simulink model "controller_v13"  (R2020b)
settings: Solver=ode4  StartTime=0.0  StopTime=inf  RelTol=1e-3
undefined symbols (not defined in the file): ctr, DiscIntNeverNeededParam, flt, IO397, mdl, rbt, rsim, som, ukf_P0_flat, ukf_prediction_time, ukf_s0, ukf_sys, ukf_use_prediction
libraries: simulink x31, slrealtimeloglib x5, slrealtimeseriallib x5, speedgoatlib_fpga_analog_io x4, slrealtimetgmanagement x3, speedgoatlib_fpga x2, speedgoatlib_fpga_dio x1, slrealtimeutilitieslib x1
(part 3 of 5)

== system controller_v13/signal generator/Drive_Signal4/AveragedAmp_filtered ==
  note: To avoid having signal "jump",
      | we want SMOOTH transitions
      | in frequency (i.e., a weighted sum
      | of current freq and freq some delta t ago)
  note: time constant 0.002sec
      | for 10kHz samping
  In1 : Inport
  Discrete Transfer Fcn : DiscreteTransferFcn  Numerator=[0.05]  Denominator=[1 -.95]
  Out1 : Outport
  wires:
  In1/1 -> Discrete Transfer Fcn/1
  Discrete Transfer Fcn/1 -> Out1/1

== system controller_v13/signal generator/Drive_Signal4/AveragedOffset_filtered ==
  note: To avoid having signal "jump",
      | we want SMOOTH transitions
      | in frequency (i.e., a weighted sum
      | of current freq and freq some delta t ago)
  note: c
  note: time constant 0.02sec
      | for 10kHz samping
  In1 : Inport
  Discrete Transfer Fcn : DiscreteTransferFcn  Numerator=[0.05]  Denominator=[1 -.95]
  Out1 : Outport
  wires:
  In1/1 -> Discrete Transfer Fcn/1
  Discrete Transfer Fcn/1 -> Out1/1

== system controller_v13/signal generator/Drive_Signal4/AveragedTau_filtered ==
  note: To avoid having signal "jump",
      | we want SMOOTH transitions
      | in frequency (i.e., a weighted sum
      | of current freq and freq some delta t ago)
  note: time constant 0.002sec
      | for 10kHz samping
  In1 : Inport
  Discrete Transfer Fcn : DiscreteTransferFcn  Numerator=[0.05]  Denominator=[1, -0.95]
  Out1 : Outport
  wires:
  In1/1 -> Discrete Transfer Fcn/1
  Discrete Transfer Fcn/1 -> Out1/1

== system controller_v13/signal generator/Drive_Signal4/SignalForRamp_binary ==
  note: Should output 1 or -1,
      | so signal ramps UP to 1
      | or DOWN to 0.
  In1 : Inport
  Add : Sum  Inputs=+-
  Compare To Zero : simulink/Logic and Bit Operations/Compare To Zero  relop=>  OutDataTypeStr=uint8  ZeroCross=off
  Constant : Constant
  Data Type Conversion : DataTypeConversion  OutDataTypeStr=double
  Gain : Gain  Gain=2
  Out1 : Outport
  wires:
  In1/1 -> Compare To Zero/1
  Compare To Zero/1 -> Data Type Conversion/1
  Gain/1 -> Add/1
  Constant/1 -> Add/2
  Add/1 -> Out1/1
  Data Type Conversion/1 -> Gain/1

== system controller_v13/signal generator/Drive_Signal4/SignalForSin_binary ==
  note: We want this to stay "high" for 1
      | second after the actual "enable"
      | is turned off...
  In1 : Inport
  Compare To Zero : simulink/Logic and Bit Operations/Compare To Zero  relop=>  OutDataTypeStr=uint8  ZeroCross=off
  Data Type Conversion : DataTypeConversion  OutDataTypeStr=double
  Out1 : Outport
  wires:
  In1/1 -> Compare To Zero/1
  Compare To Zero/1 -> Data Type Conversion/1
  Data Type Conversion/1 -> Out1/1

== system controller_v13/signal generator/Drive_Signal4/Subsystem ==
  note: positive value pushes the left wing forward
  split cycle mu : Inport
  In2 : Inport  Port=2
  1-mu : Sum  Inputs=+-
  2f : Gain  Gain=2
  2nd harmonic : Trigonometry  OutputSignalType=real
  2pi : Gain  Gain=2*pi
  Abs1 : Abs
  Add : Sum
  Constant : Constant
  combined sines : Sum
  deg to rad : Gain  Gain=pi/180
  f : Gain  Gain=-1
  first harmonic : Trigonometry  OutputSignalType=real
  omega*t : DiscreteIntegrator  SampleTime=-1  ICPrevOutput=DiscIntNeverNeededParam  ICPrevScaledInput=DiscIntNeverNeededParam
  phase offset : Constant  Value=0
  signal with gain1 : Product  RndMeth=Zero
  signal with gain2 : Product  RndMeth=Zero
  split cycle signal : Outport
  wires:
  2f/1 -> 2nd harmonic/1
  first harmonic/1 -> signal with gain1/2
  Constant/1 -> 1-mu/1
  split cycle mu/1 -> f/1, Abs1/1
  1-mu/1 -> signal with gain1/1
  2nd harmonic/1 -> signal with gain2/2
  signal with gain1/1 -> combined sines/1
  signal with gain2/1 -> combined sines/2
  combined sines/1 -> split cycle signal/1
  f/1 -> signal with gain2/1
  Abs1/1 -> 1-mu/2
  In2/1 -> 2pi/1
  2pi/1 -> omega*t/1
  omega*t/1 -> Add/2
  Add/1 -> first harmonic/1, 2f/1
  phase offset/1 -> deg to rad/1
  deg to rad/1 -> Add/1

== system controller_v13/Adaptive Controller/adaptive system/integrator/safety2 ==
  In1 : Inport
  Compare To Constant1 : simulink/Logic and Bit Operations/Compare To Constant  relop=<=  const=inf  OutDataTypeStr=uint8
  Switch1 : Switch  Threshold=0.5
  zero1 : Constant  Value=0
  Out1 : Outport
  wires:
  In1/1 -> Switch1/1, Compare To Constant1/1
  Compare To Constant1/1 -> Switch1/2
  zero1/1 -> Switch1/3
  Switch1/1 -> Out1/1

== system controller_v13/Adaptive Controller/adaptive system/integrator/start ramp ==
  0.8 : Constant  Value=mdl.s_delay
  2 : Constant  Value=mdl.i_delay
  Add1 : Sum
  Add2 : Sum  Inputs=+-
  Compare To Zero : simulink/Logic and Bit Operations/Compare To Zero  relop=>  OutDataTypeStr=uint8  ZeroCross=off
  Data Type Conversion : DataTypeConversion
  constant : Constant
  counter : DiscreteIntegrator  gainval=1  SampleTime=-1  UpperSaturationLimit=1  LowerSaturationLimit=0  ICPrevOutput=DiscIntNeverNeededParam  ICPrevScaledInput=DiscIntNeverNeededParam
  saturation ramp : DiscreteIntegrator  gainval=5  SampleTime=-1  LimitOutput=on  UpperSaturationLimit=1  LowerSaturationLimit=-1  ICPrevOutput=DiscIntNeverNeededParam  ICPrevScaledInput=DiscIntNeverNeededParam
  Out1 : Outport
  wires:
  constant/1 -> counter/1
  2/1 -> Add1/1
  0.8/1 -> Add1/2
  counter/1 -> Add2/1
  Add1/1 -> Add2/2
  Add2/1 -> Compare To Zero/1
  Compare To Zero/1 -> Data Type Conversion/1
  saturation ramp/1 -> Out1/1
  Data Type Conversion/1 -> saturation ramp/1

== system controller_v13/Adaptive Controller/observer/Linear Observer (ICRA'23)/Rotaion ==
  Euler : Inport
  Rotation Matrix : MATLAB Function  TreatAsAtomicUnit=on
  Rotation Matrix1 : MATLAB Function  TreatAsAtomicUnit=on
  filtered derivative : Subsystem
  R : Outport
  Rdot : Outport  Port=2
  Omega : Outport  Port=3
  wires:
  Rotation Matrix/1(R) -> filtered derivative/1(In1), Rotation Matrix1/1(R), R/1
  Euler/1 -> Rotation Matrix/1(euler_angles)
  filtered derivative/1(Out1) -> Rotation Matrix1/2(Rdot), Rdot/1
  Rotation Matrix1/1(w) -> Omega/1

== system controller_v13/Adaptive Controller/observer/Linear Observer (ICRA'23)/lateral KF observer ==
  note: x_hat_pred
  R : Inport
  f_cmd : Inport  Port=2
  xyz : Inport  Port=3
  Delay : Delay  DelayLength=1  InitialCondition=zeros(3,1)
  Delay1 : Delay  DelayLength=1  InitialCondition=zeros(3,1)  SampleTime=mdl.T
  Delay2 : Delay  DelayLength=1  InitialCondition=1
  Scope1 : Scope
  Scope2 : Scope
  Translational Dynamics & Kinamatics Lin Obs : MATLAB Function  TreatAsAtomicUnit=on
  r : Outport
  r_dot : Outport  Port=2
  r_dotdot : Outport  Port=3
  wires:
  R/1 -> Translational Dynamics & Kinamatics Lin Obs/1(R)
  Translational Dynamics & Kinamatics Lin Obs/3(acc_hat) -> r_dotdot/1
  Delay/1 -> Translational Dynamics & Kinamatics Lin Obs/5("vel_hat ")
  xyz/1 -> Translational Dynamics & Kinamatics Lin Obs/3(meas_pos)
  Translational Dynamics & Kinamatics Lin Obs/2(vel_hat) -> Scope1/1, r_dot/1, Delay/1
  Translational Dynamics & Kinamatics Lin Obs/1(pos_hat) -> Delay1/1, Scope2/1, r/1
  f_cmd/1 -> Translational Dynamics & Kinamatics Lin Obs/2(f_cmd)
  Delay1/1 -> Translational Dynamics & Kinamatics Lin Obs/4("pos_hat ")
  Translational Dynamics & Kinamatics Lin Obs/4(id_out) -> Delay2/1
  Delay2/1 -> Translational Dynamics & Kinamatics Lin Obs/6(id_in)

== system controller_v13/Adaptive Controller/observer/Linear Observer (ICRA'23)/lateral observer ==
  XYZ : Inport
  derivative filter : simulink/Discrete/Transfer Fcn Lead or Lag  PoleZ=mdl.zf1  ZeroZ=1  ICPrevOutput=0.0  ICPrevInput=0.0  DoSatur=off
      settings: SourceProductBaseCode=SL
  derivative filter1 : simulink/Discrete/Transfer Fcn Lead or Lag  PoleZ=mdl.zf2  ZeroZ=1  ICPrevOutput=0.0  ICPrevInput=0.0  DoSatur=off
      settings: SourceProductBaseCode=SL
  derivative filter2 : simulink/Discrete/Transfer Fcn Lead or Lag  PoleZ=mdl.zf2  ZeroZ=1  ICPrevOutput=0.0  ICPrevInput=0.0  DoSatur=off
      settings: SourceProductBaseCode=SL
  lat_s : Gain  Gain=mdl.f1
  lat_s2 : Gain  Gain=mdl.f2
  lat_s2_ : Gain  Gain=mdl.f2
  saturation : Subsystem
  r : Outport
  r_dot : Outport  Port=2
  r_dotdot : Outport  Port=3
  wires:
  derivative filter1/1 -> derivative filter2/1
  derivative filter/1 -> lat_s/1
  XYZ/1 -> derivative filter/1, derivative filter1/1, r/1
  derivative filter2/1 -> lat_s2/1
  lat_s/1 -> r_dot/1
  lat_s2/1 -> lat_s2_/1
  lat_s2_/1 -> saturation/1(In1)
  saturation/1(Out1) -> r_dotdot/1

== system controller_v13/Adaptive Controller/observer/UKF/UKF ==
  r_in : Inport
  euler : Inport  Port=2
  r_dot_in : Inport  Port=3
  omega_in : Inport  Port=4
  f_cmd : Inport  Port=5
  tau_cmd_x : Inport  Port=6
  tau_cmd_y : Inport  Port=7
  To Workspace1 : ToWorkspace  VariableName=ukf_z_in  SaveFormat=Timeseries  SampleTime=-1
  To Workspace2 : ToWorkspace  VariableName=ukf_s  SaveFormat=Timeseries  SampleTime=-1
  To Workspace3 : ToWorkspace  VariableName=ukf_f_cmd  SaveFormat=Timeseries  SampleTime=-1
  To Workspace4 : ToWorkspace  VariableName=ukf_tau_cmd_x  SaveFormat=Timeseries  SampleTime=-1
  To Workspace5 : ToWorkspace  VariableName=ukf_tau_cmd_y  SaveFormat=Timeseries  SampleTime=-1
  UKF_inner : Subsystem
  euler to quat : MATLAB Function  TreatAsAtomicUnit=on
  pack measurement vector : MATLAB Function  TreatAsAtomicUnit=on
  quaternion to rotation matrix : MATLAB Function  TreatAsAtomicUnit=on
  unpack state vector : MATLAB Function  TreatAsAtomicUnit=on
  r_out : Outport
  r_dot_out : Outport  Port=2
  R_out : Outport  Port=3
  omega_out : Outport  Port=4
  wires:
  r_in/1 -> pack measurement vector/1(r)
  r_dot_in/1 -> pack measurement vector/3(r_dot)
  omega_in/1 -> pack measurement vector/4(omega)
  f_cmd/1 -> UKF_inner/2(f_cmd), To Workspace3/1
  tau_cmd_x/1 -> UKF_inner/3(tau_cmd_x), To Workspace4/1
  tau_cmd_y/1 -> To Workspace5/1, UKF_inner/4(tau_cmd_y)
  euler to quat/1(q) -> pack measurement vector/2(q)
  quaternion to rotation matrix/1(R_flat) -> R_out/1
  euler/1 -> euler to quat/1(euler_angles)
  pack measurement vector/1(z_raw) -> UKF_inner/1(z_raw), To Workspace1/1
  unpack state vector/1(r) -> r_out/1
  unpack state vector/2(q) -> quaternion to rotation matrix/1(q)
  unpack state vector/3(r_dot) -> r_dot_out/1
  unpack state vector/4(omega) -> omega_out/1
  UKF_inner/1(s_out) -> unpack state vector/1(s), To Workspace2/1

== system controller_v13/Adaptive Controller/observer/UKF/UKF1 ==
  r_in : Inport
  R_in : Inport  Port=2
  f_cmd : Inport  Port=3
  tau_cmd_x : Inport  Port=4
  tau_cmd_y : Inport  Port=5
  s_prediciton_time : Inport  Port=6
  R_flat to quat : MATLAB Function  TreatAsAtomicUnit=on
  Switch : Switch  Criteria=u2 > Threshold
  To Workspace1 : ToWorkspace  VariableName=ukf_z_in  SaveFormat=Timeseries  SampleTime=-1
  To Workspace14 : ToWorkspace  VariableName=ukf_s_prediction_out  SaveFormat=Timeseries  SampleTime=-1
  To Workspace2 : ToWorkspace  VariableName=ukf_s  SaveFormat=Timeseries  SampleTime=-1
  To Workspace3 : ToWorkspace  VariableName=ukf_f_cmd  SaveFormat=Timeseries  SampleTime=-1
  To Workspace4 : ToWorkspace  VariableName=ukf_tau_cmd_x  SaveFormat=Timeseries  SampleTime=-1
  To Workspace5 : ToWorkspace  VariableName=ukf_tau_cmd_y  SaveFormat=Timeseries  SampleTime=-1
  UKF_inner : Subsystem
  pack measurement vector : MATLAB Function  TreatAsAtomicUnit=on
  quaternion to rotation matrix : MATLAB Function  TreatAsAtomicUnit=on
  unpack state : MATLAB Function  TreatAsAtomicUnit=on
  use prediction : Constant  Value=ukf_use_prediction
  r_out : Outport
  r_dot_out : Outport  Port=2
  R_out : Outport  Port=3
  omega_out : Outport  Port=4
  F_ext : Outport  Port=5
  tau_ext : Outport  Port=6
  wires:
  r_in/1 -> pack measurement vector/1(r)
  f_cmd/1 -> To Workspace3/1, UKF_inner/2(f_cmd)
  tau_cmd_x/1 -> To Workspace4/1, UKF_inner/3(tau_cmd_x)
  tau_cmd_y/1 -> To Workspace5/1, UKF_inner/4(tau_cmd_y)
  R_flat to quat/1(q) -> pack measurement vector/2(q)
  quaternion to rotation matrix/1(R_flat) -> R_out/1
  pack measurement vector/1(z_raw) -> To Workspace1/1, UKF_inner/1(z_raw)
  unpack state/1(r) -> r_out/1
  unpack state/2(q) -> quaternion to rotation matrix/1(q)
  unpack state/3(r_dot) -> r_dot_out/1
  unpack state/4(omega) -> omega_out/1
  R_in/1 -> R_flat to quat/1(R_flat)
  s_prediciton_time/1 -> UKF_inner/5(s_prediction_time)
  Switch/1 -> unpack state/1(s)
  use prediction/1 -> Switch/2
  UKF_inner/2(s_out) -> To Workspace2/1, Switch/3
  UKF_inner/1(s_prediction_out) -> To Workspace14/1, Switch/1
  unpack state/5(F_ext) -> F_ext/1
  unpack state/6(tau_ext) -> tau_ext/1

== system controller_v13/Adaptive Controller/observer/UKF/UKF2 ==
  r_in : Inport
  euler : Inport  Port=2
  r_dot_in : Inport  Port=3
  omega_in : Inport  Port=4
  f_cmd : Inport  Port=5
  tau_cmd_x : Inport  Port=6
  tau_cmd_y : Inport  Port=7
  To Workspace1 : ToWorkspace  VariableName=ukf_z_in  SaveFormat=Timeseries  SampleTime=-1
  To Workspace2 : ToWorkspace  VariableName=ukf_s  SaveFormat=Timeseries  SampleTime=-1
  To Workspace3 : ToWorkspace  VariableName=ukf_f_cmd  SaveFormat=Timeseries  SampleTime=-1
  To Workspace4 : ToWorkspace  VariableName=ukf_tau_cmd_x  SaveFormat=Timeseries  SampleTime=-1
  To Workspace5 : ToWorkspace  VariableName=ukf_tau_cmd_y  SaveFormat=Timeseries  SampleTime=-1
  UKF_inner : Subsystem
  euler to quat : MATLAB Function  TreatAsAtomicUnit=on
  pack measurement vector : MATLAB Function  TreatAsAtomicUnit=on
  quaternion to rotation matrix : MATLAB Function  TreatAsAtomicUnit=on
  unpack state vector : MATLAB Function  TreatAsAtomicUnit=on
  r_out : Outport
  r_dot_out : Outport  Port=2
  R_out : Outport  Port=3
  omega_out : Outport  Port=4
  wires:
  r_in/1 -> pack measurement vector/1(r)
  r_dot_in/1 -> pack measurement vector/3(r_dot)
  omega_in/1 -> pack measurement vector/4(omega)
  f_cmd/1 -> UKF_inner/2(f_cmd), To Workspace3/1
  tau_cmd_x/1 -> UKF_inner/3(tau_cmd_x), To Workspace4/1
  tau_cmd_y/1 -> To Workspace5/1, UKF_inner/4(tau_cmd_y)
  euler to quat/1(q) -> pack measurement vector/2(q)
  quaternion to rotation matrix/1(R_flat) -> R_out/1
  euler/1 -> euler to quat/1(euler_angles)
  pack measurement vector/1(z_raw) -> UKF_inner/1(z_raw), To Workspace1/1
  unpack state vector/1(r) -> r_out/1
  unpack state vector/2(q) -> quaternion to rotation matrix/1(q)
  unpack state vector/3(r_dot) -> r_dot_out/1
  unpack state vector/4(omega) -> omega_out/1
  UKF_inner/1(s_out) -> unpack state vector/1(s), To Workspace2/1

== system controller_v13/Adaptive Controller/observer/UKF/lateral observer ==
  XYZ : Inport
  derivative filter : simulink/Discrete/Transfer Fcn Lead or Lag  PoleZ=mdl.zf1  ZeroZ=1  ICPrevOutput=0.0  ICPrevInput=0.0  DoSatur=off
      settings: SourceProductBaseCode=SL
  derivative filter1 : simulink/Discrete/Transfer Fcn Lead or Lag  PoleZ=mdl.zf2  ZeroZ=1  ICPrevOutput=0.0  ICPrevInput=0.0  DoSatur=off
      settings: SourceProductBaseCode=SL
  derivative filter2 : simulink/Discrete/Transfer Fcn Lead or Lag  PoleZ=mdl.zf2  ZeroZ=1  ICPrevOutput=0.0  ICPrevInput=0.0  DoSatur=off
      settings: SourceProductBaseCode=SL
  lat_s : Gain  Gain=mdl.f1
  lat_s2 : Gain  Gain=mdl.f2
  lat_s2_ : Gain  Gain=mdl.f2
  saturation : Subsystem
  r : Outport
  r_dot : Outport  Port=2
  r_dotdot : Outport  Port=3
  wires:
  derivative filter1/1 -> derivative filter2/1
  derivative filter/1 -> lat_s/1
  XYZ/1 -> derivative filter/1, derivative filter1/1, r/1
  derivative filter2/1 -> lat_s2/1
  lat_s/1 -> r_dot/1
  lat_s2/1 -> lat_s2_/1
  lat_s2_/1 -> saturation/1(In1)
  saturation/1(Out1) -> r_dotdot/1

== system controller_v13/Adaptive Controller/observer/Linear Observer (ICRA'23)/Rotaion/filtered derivative ==
  In1 : Inport
  att_s : Gain  Gain=mdl.f1
  filtered derivative : simulink/Discrete/Transfer Fcn Lead or Lag  PoleZ=mdl.zf1  ZeroZ=1  ICPrevOutput=0.0  ICPrevInput=0.0  DoSatur=off
      settings: SourceProductBaseCode=SL
  low pass3 : DiscreteTransferFcn  Numerator=mdl.vlp.n  Denominator=mdl.vlp.d
  Out1 : Outport
  wires:
  filtered derivative/1 -> low pass3/1
  att_s/1 -> filtered derivative/1
  In1/1 -> att_s/1
  low pass3/1 -> Out1/1

== system controller_v13/Adaptive Controller/observer/Linear Observer (ICRA'23)/lateral observer/saturation ==
  In1 : Inport
  MinMax2 : MinMax  Inputs=2
  MinMax3 : MinMax  Function=max  Inputs=2
  lw1 : Constant  Value=-mdl.fd_lim
  up1 : Constant  Value=mdl.fd_lim
  Out1 : Outport
  wires:
  In1/1 -> MinMax2/2
  up1/1 -> MinMax2/1
  lw1/1 -> MinMax3/1
  MinMax2/1 -> MinMax3/2
  MinMax3/1 -> Out1/1

== system controller_v13/Adaptive Controller/observer/UKF/UKF/UKF_inner ==
  z_raw : Inport
  f_cmd : Inport  Port=2
  tau_cmd_x : Inport  Port=3
  tau_cmd_y : Inport  Port=4
  Delay : Delay  DelayLength=1  InitialCondition="reshape((   diag(vertcat(   1e-4 * ones(12,1),   [0.107 * 7.2e-4; 0.107 * 7.2e-4; 0.107 * 7.2e-4],   [1.1e-21; 1.1e-21; 1e-21]   ))   )',   1,   []   )'"  SampleTime=mdl.T
  Delay1 : Delay  DelayLength=1  InitialCondition=vertcat( [0;0;0], [1;0;0;0], [0;0;0], [0;0;0], [0.981 * 7.2e-4; 0.981 * 7.2e-4; 0.981 * 7.2e-4], [5e-6;5e-6;0] )  SampleTime=mdl.T
  Delay2 : Delay  DelayLength=1  InitialCondition=zeros(13,1)  SampleTime=mdl.T
  Delay3 : Delay  DelayLength=1  InitialCondition=0  SampleTime=mdl.T
  To Workspace3 : ToWorkspace  VariableName=ukf_P_flats  SaveFormat=Timeseries  SampleTime=-1
  UKF update then predict : MATLAB Function  TreatAsAtomicUnit=on  mask{sys=ukf_sys}
  s_out : Outport
  wires:
  z_raw/1 -> UKF update then predict/1(z_raw), Delay2/1
  f_cmd/1 -> UKF update then predict/3(f_cmd)
  tau_cmd_x/1 -> UKF update then predict/4(tau_cmd_x)
  tau_cmd_y/1 -> UKF update then predict/5(tau_cmd_y)
  UKF update then predict/1(s_out) -> s_out/1, Delay1/1
  UKF update then predict/2(P_out_flat) -> Delay/1
  Delay/1 -> UKF update then predict/7(P_in_flat), To Workspace3/1
  Delay1/1 -> UKF update then predict/6(s_in)
  Delay2/1 -> UKF update then predict/2(z_raw_prev)
  UKF update then predict/3(is_init_out) -> Delay3/1
  Delay3/1 -> UKF update then predict/8(is_init_in)

== system controller_v13/Adaptive Controller/observer/UKF/UKF1/UKF_inner ==
  z_raw : Inport
  f_cmd : Inport  Port=2
  tau_cmd_x : Inport  Port=3
  tau_cmd_y : Inport  Port=4
  s_prediction_time : Inport  Port=5
  Delay : Delay  DelayLength=1  InitialCondition=ukf_P0_flat  SampleTime=mdl.T
  Delay1 : Delay  DelayLength=1  InitialCondition=ukf_s0  SampleTime=mdl.T
  Delay2 : Delay  DelayLength=1  InitialCondition=[0,0,0, 1,0,0,0,0, 0,0,0, 0,0]'  SampleTime=mdl.T
  Delay3 : Delay  DelayLength=1  InitialCondition=0  SampleTime=mdl.T
  Scope : Scope
  Terminator : Terminator
  To Workspace3 : ToWorkspace  VariableName=ukf_P_flats  SaveFormat=Timeseries  SampleTime=-1
  UKF update then predict : MATLAB Function  TreatAsAtomicUnit=on  mask{sys=ukf_sys}
  bee cov to SI cov : MATLAB Function  TreatAsAtomicUnit=on
  bee units to SI : MATLAB Function  TreatAsAtomicUnit=on
  bee units to SI1 : MATLAB Function  TreatAsAtomicUnit=on
  s_prediction_out : Outport
  s_out : Outport  Port=2
  wires:
  z_raw/1 -> Delay2/1, UKF update then predict/1(z_raw)
  f_cmd/1 -> UKF update then predict/3(f_cmd)
  tau_cmd_x/1 -> UKF update then predict/4(tau_cmd_x)
  tau_cmd_y/1 -> UKF update then predict/5(tau_cmd_y)
  UKF update then predict/1(s_out) -> Delay1/1, bee units to SI/1(s_bee)
  UKF update then predict/2(P_out_flat) -> Delay/1
  Delay/1 -> UKF update then predict/7(P_in_flat), bee cov to SI cov/1(P_flat_bee)
  Delay1/1 -> UKF update then predict/6(s_in)
  Delay2/1 -> UKF update then predict/2(z_raw_prev)
  UKF update then predict/3(is_init_out) -> Delay3/1
  Delay3/1 -> UKF update then predict/8(is_init_in)
  UKF update then predict/4(s_out_pre) -> Terminator/1
  bee units to SI/1(s_si) -> s_out/1  "UKF states"
  bee cov to SI cov/1(P_flat_si) -> To Workspace3/1
  UKF update then predict/5(s_prediction_out) -> bee units to SI1/1(s_bee)
  s_prediction_time/1 -> UKF update then predict/9(s_prediction_time)
  bee units to SI1/1(s_si) -> s_prediction_out/1  "UKF states prediction"
  UKF update then predict/6(md) -> Scope/1  "mahalnobis_distance"

== system controller_v13/Adaptive Controller/observer/UKF/UKF2/UKF_inner ==
  z_raw : Inport
  f_cmd : Inport  Port=2
  tau_cmd_x : Inport  Port=3
  tau_cmd_y : Inport  Port=4
  Delay : Delay  DelayLength=1  InitialCondition="reshape((   diag(vertcat(   1e-4 * ones(12,1),   [0.107 * 7.2e-4; 0.107 * 7.2e-4; 0.107 * 7.2e-4],   [1.1e-21; 1.1e-21; 1e-21]   ))   )',   1,   []   )'"  SampleTime=mdl.T
  Delay1 : Delay  DelayLength=1  InitialCondition=vertcat( [0;0;0], [1;0;0;0], [0;0;0], [0;0;0], [0.981 * 7.2e-4; 0.981 * 7.2e-4; 0.981 * 7.2e-4], [5e-6;5e-6;0] )  SampleTime=mdl.T
  Delay2 : Delay  DelayLength=1  InitialCondition=zeros(13,1)  SampleTime=mdl.T
  Delay3 : Delay  DelayLength=1  InitialCondition=0  SampleTime=mdl.T
  To Workspace3 : ToWorkspace  VariableName=ukf_P_flats  SaveFormat=Timeseries  SampleTime=-1
  UKF update then predict : MATLAB Function  TreatAsAtomicUnit=on  mask{sys=ukf_sys}
  s_out : Outport
  wires:
  z_raw/1 -> UKF update then predict/1(z_raw), Delay2/1
  f_cmd/1 -> UKF update then predict/3(f_cmd)
  tau_cmd_x/1 -> UKF update then predict/4(tau_cmd_x)
  tau_cmd_y/1 -> UKF update then predict/5(tau_cmd_y)
  UKF update then predict/1(s_out) -> s_out/1, Delay1/1
  UKF update then predict/2(P_out_flat) -> Delay/1
  Delay/1 -> UKF update then predict/7(P_in_flat), To Workspace3/1
  Delay1/1 -> UKF update then predict/6(s_in)
  Delay2/1 -> UKF update then predict/2(z_raw_prev)
  UKF update then predict/3(is_init_out) -> Delay3/1
  Delay3/1 -> UKF update then predict/8(is_init_in)

== system controller_v13/Adaptive Controller/observer/UKF/lateral observer/saturation ==
  In1 : Inport
  MinMax2 : MinMax  Inputs=2
  MinMax3 : MinMax  Function=max  Inputs=2
  lw1 : Constant  Value=-mdl.fd_lim
  up1 : Constant  Value=mdl.fd_lim
  Out1 : Outport
  wires:
  In1/1 -> MinMax2/2
  up1/1 -> MinMax2/1
  lw1/1 -> MinMax3/1
  MinMax2/1 -> MinMax3/2
  MinMax3/1 -> Out1/1

== matlab function controller_v13/Adaptive Controller/observer/Linear Observer (ICRA'23)/Rotaion/Rotation Matrix ==
  data: euler_angles input; R output
function R = fcn(euler_angles)
%#codegen

eu_x = euler_angles(1);
eu_y = euler_angles(2);
eu_z = euler_angles(3);

R = [cos(eu_y)*cos(eu_z); -cos(eu_y)*sin(eu_z); sin(eu_y); ...
    cos(eu_x)*sin(eu_z)+sin(eu_x)*sin(eu_y)*cos(eu_z); cos(eu_x)*cos(eu_z)-sin(eu_x)*sin(eu_y)*sin(eu_z); -sin(eu_x)*cos(eu_y); ...
    sin(eu_x)*sin(eu_z)-cos(eu_x)*sin(eu_y)*cos(eu_z); sin(eu_x)*cos(eu_z)+cos(eu_x)*sin(eu_y)*sin(eu_z); cos(eu_x)*cos(eu_y)];
% R is 9x1

== matlab function controller_v13/Adaptive Controller/attitude and thrust controller1/Thrust Controller ==
  data: r input; F output size=1; r_dot input; r_dotdot input; R input; Omega input; rd input; rd_d input; rd_dd input; rd_ddd input; rd_dddd input; int_e input; mdl parameter; alt_e output size=1; ctr parameter
function [F, alt_e] = fcn(r, r_dot, r_dotdot, R, Omega, rd,rd_d,rd_dd,rd_ddd,rd_dddd, int_e, mdl, ctr)
%#codegen

%% init
R11 = R(1);
R12 = R(2);
R13 = R(3);
R21 = R(4);
R22 = R(5);
R23 = R(6);
R31 = R(7);
R32 = R(8);
R33 = R(9);


F = rd_dd(3) - ctr.gain.al1*( r_dot(3)-rd_d(3) ) - ctr.gain.al0*( r(3)-rd(3) );
% F = 0 - ctr.gain.al1*( r_dot(3)) - ctr.gain.al0*( r(3)-ctr.setpoint.z );
F = mdl.g + F + ctr.gain.ali*int_e(4);
F = F/R33;
F = max(min(F, mdl.g+4), mdl.g-3.0); % during hovering.

alt_e = -( r(3)-rd(3) )/R33;
% alt_e = -( r(3)- ctr.setpoint.z )/R33;
end

== matlab function controller_v13/Adaptive Controller/adaptive setpoint rd ==
  data: rd output; rd_d output; rd_dd output; rd_ddd output; rd_dddd output; time input; r input; r_d input; landing input; som_ph input; ctr parameter; som parameter; mdl parameter
function [rd,rd_d,rd_dd,rd_ddd,rd_dddd] = fcn(time, r, r_d, landing,som_ph, ctr, som, mdl)
%#codegen

rd = [ctr.setpoint.x; ctr.setpoint.y; ctr.setpoint.z];
rd_d = zeros(3,1);
rd_dd = zeros(3,1);
rd_ddd = zeros(3,1);
rd_dddd = zeros(3,1);

if time <= mdl.i_delay
    rd_z = 0;
    rd   = [ctr.setpoint.x; ctr.setpoint.y; rd_z];
end

% takeoff
if ctr.takeoff.en
    if time > mdl.i_delay && time < (mdl.i_delay+ctr.takeoff.time)
        rd_z = ctr.takeoff.height + (((ctr.setpoint.z-ctr.takeoff.height)/ctr.takeoff.time)*(time-mdl.i_delay));
        if rd_z > ctr.setpoint.z
            rd_z = ctr.setpoint.z;
        end
        rd   = [ctr.setpoint.x; ctr.setpoint.y; rd_z];
    end
end

% planned landing 
if ctr.landing.en
    if time > (mdl.rt-ctr.landing.time)
        rd_z = ctr.setpoint.z-(((ctr.setpoint.z-ctr.landing.height)/ctr.landing.time)*(time-mdl.rt+ctr.landing.time));
        if rd_z < ctr.landing.height
            rd_z = ctr.landing.height;
        end
        rd   = [ctr.setpoint.x; ctr.setpoint.y; rd_z];
    end
end

% forced landing
if landing
    rd_z = 0.02;
    rd   = [ctr.setpoint.x; ctr.setpoint.y; rd_z];
end


% somersault
if som.en
    if time > som.t_start + som.t_rise + som.t_acc + som.t_dcc + som.t_rec
        % % afterwards 
        %dt = som.t_start + som.t_rise + som.t_acc + som.t_dcc + som.t_rec - time;
        %rd = rd + dt*(r-rd);
    elseif time > som.t_start + som.t_rise + som.t_acc + som.t_dcc
        % recovery
        dt = som.t_start + som.t_rise + som.t_acc + som.t_dcc + som.t_rec - time;
        rd = rd + (dt/som.t_rec)*(r-rd);
        rd_d = rd_d + 0.5*(dt/som.t_rec)*(r_d-rd_d);
        rd(1) = min(max(rd(1),-0.25),0.25); % 25 cm envelope
        rd(2) = min(max(rd(2),-0.25),0.25); % 25 cm envelope
        rd(3) = max(rd(3),0.02); % min altitude setpoint.
    end
end


end

== matlab function controller_v13/Force//Torque to Trajectory Specs/nominal desired voltage/force to voltage (hovering) /MATLAB Function ==
  data: Vi input; Vo output; mdl parameter
function Vo = fcn(Vi,mdl)
%old script
% if max(Vi)>mdl.max_v
%     Vo = Vi * mdl.max_v/max(Vi);
%     % scale down all votages if one exceeds the max limit.
% else
%     Vo = Vi;
% end

%new change (modify max_v to a vector so each DEA has its own max)
% scale_down_ratio_vec = Vi ./ mdl.max_v_vec;
% scale_down_ratio = max(scale_down_ratio_vec);
% bool_scale_down = scale_down_ratio>1;
% 
% if bool_scale_down
%    Vo = Vi/scale_down_ratio;
% else
%    Vo = Vi; 
% end

min_v_vec = mdl.hovering_vec -150;
scale_down_ratio_vec = (Vi-min_v_vec)./(mdl.max_v_vec-min_v_vec);

scale_down_ratio = max(scale_down_ratio_vec);
bool_scale_down = scale_down_ratio>1;

if bool_scale_down
    Vo = min_v_vec + (Vi - min_v_vec)./scale_down_ratio;	
else
	  Vo = Vi; 
end


%extra layer of safety
for i=1:length(Vo)
	Vo(i) = min(Vo(i),mdl.max_v_vec(i));
end

== matlab function controller_v13/Adaptive Controller/somersault_phase ==
  data: som_phase output; time input; mdl parameter; som parameter
function som_phase  = fcn(time, mdl, som)
%#codegen

som_phase = 0;  % during a normal flight
if som.en
    if time > som.t_start + som.t_rise + som.t_acc + som.t_dcc + som.t_rec
        som_phase = 0;  % afterwards
    elseif time > som.t_start + som.t_rise + som.t_acc + som.t_dcc
        som_phase = 4;  % recovery
    elseif time > som.t_start + som.t_rise + som.t_acc
        som_phase = 3;  % rolling, second half.
    elseif time > som.t_start + som.t_rise
        som_phase = 2;  % rolling, first half.
    elseif time > som.t_start
        som_phase = 1;  % gaining altitude
    end
end

== matlab function controller_v13/Force//Torque to Trajectory Specs/nominal desired voltage/force to voltage flipping/MATLAB Function ==
  data: Vi input; Vo output; mdl parameter
function Vo = fcn(Vi,mdl)
%old script
% if max(Vi)>mdl.max_v
%     Vo = Vi * mdl.max_v/max(Vi);
%     % scale down all votages if one exceeds the max limit.
% else
%     Vo = Vi;
% end

%new change (modify max_v to a vector so each DEA has its own max)
scale_down_ratio_vec = Vi ./ mdl.max_v_vec;
scale_down_ratio = max(scale_down_ratio_vec);
bool_scale_down = scale_down_ratio>1;

if bool_scale_down
   Vo = Vi/scale_down_ratio;
else
   Vo = Vi; 
end

== matlab function controller_v13/smothing/smoothing ==
  data: time input; out_amp output; amp input; amp2 input; som parameter
function out_amp  = fcn(time,amp,amp2,som)
%#codegen

alp = 1;
if time > som.t_start + som.t_rise + som.t_acc + som.t_dcc + som.t_rec
    alp = 1;  % afterwards
elseif time > som.t_start
    alp = som.filter.alp;
end
% set en = 0 if the robot goes out of the safe envelope.
out_amp = som.filter.alp*amp + (1-som.filter.alp)*amp2;

== matlab function controller_v13/Adaptive Controller/saturation ==
  data: x_roll input; X_roll output size=1; y_pitch input; z_yaw input; Y_pitch output size=1; Z_yaw output size=1; Th input; Force output size=1; rbt parameter; ctr parameter; som_phase input; som parameter; exitflag output
function [X_roll, Y_pitch, Z_yaw, Force, exitflag] = fcn(x_roll, y_pitch, z_yaw, Th, rbt, ctr, som_phase, som)
%#codegen
X_roll = 0;
Y_pitch = 0;
Z_yaw = 0;
Force = 0;

if ~ctr.adaptive_saturation.enable
    X_roll = max(min(x_roll, ctr.lim.taux), -ctr.lim.taux);
    %X_roll = x_roll;
    Y_pitch = max(min(y_pitch, ctr.lim.tauy), -ctr.lim.tauy);
    %Y_pitch = y_pitch;
    Z_yaw = max(min(z_yaw, ctr.lim.tauz), -ctr.lim.tauz);
    
    Force = Th*rbt.m;
    exitflag = 0;
else
    % adaptive saturation strategy
    [X_roll, Y_pitch, Force, exitflag] = adaptive_saturation(x_roll, y_pitch, Th*rbt.m, rbt, ctr);
    
    % 
  
    Z_yaw = 0; % max(min(z_yaw, ctr.lim.tauz), -ctr.lim.tauz);

end

% F is already checked for saturation, but still needs to be converted into
% Newton

%% Roll torque management (somersault)
if som_phase == 2
    X_roll = som.roll_mag; % torque in SI
    Y_pitch = 0;  % to turn of the pitch control
elseif som_phase == 3
    X_roll = -som.roll_mag; % torque in SI
    Y_pitch = 0;  % to turn of the pitch control
end
    
%% Thrust management
% thrust is not controlled during the flipping maneuver (the output here will be overridden in the mapping).

== matlab function controller_v13/Force//Torque to Trajectory Specs/force//torque to module thrust/mapping scheme (flipping compataible) ==
  data: time input; module_f output; inputs input; rbt parameter; som parameter; mdl parameter
function module_f  = fcn(time, inputs, rbt, som, mdl)

% somersault
if som.en
    if time > som.t_start + som.t_rise + som.t_acc + som.t_dcc+som.t_rec % after recovery
        %
    elseif time > som.t_start + som.t_rise + som.t_acc + som.t_dcc % recovery
        %inputs(1) = rbt.m*(mdl.g*(som.thrust_f+0.2));
    elseif time > som.t_start + som.t_rise % rolling, first half+second half.
        % priortize the roll torque and ensure non-negative forces.
        inputs(1) = 0;
    elseif time > som.t_start
        inputs(1) = rbt.m*(mdl.g*som.thrust_f); % during the t rise.                
    end
end

% torque/thrust to unit force mapping
if rbt.til == 0
    module_f = rbt.Apinv * inputs(1:3); % original mapping
elseif rbt.til > 0
    module_f = rbt.A2inv * inputs;
else
    module_f = [0 0 0 0]';
end

% safety
if min(module_f) < 0
    module_f = module_f - min(module_f); % this ensure positive module forces
end

end

== matlab function controller_v13/Adaptive Controller/adaptive system/integrator/initial guess ==
  data: i_e input; int_e output; tor_off input; th_off input; tor_inte output; th_inte output; ctr parameter; rbt parameter; mdl parameter
function [int_e, tor_inte, th_inte] = fcn(i_e, tor_off, th_off, ctr, rbt, mdl)
%#codegen

tor_inte = zeros(3,1);
int_e    = zeros(4,1);

int_e(1) = i_e(1)+tor_off(1);
int_e(2) = i_e(2)+tor_off(2);
int_e(3) = i_e(3)+tor_off(3);
int_e(4) = i_e(4)+th_off;

tor_inte(1) = int_e(1)*ctr.gain.ati*rbt.ixx/mdl.g;
tor_inte(2) = int_e(2)*ctr.gain.ati*rbt.iyy/mdl.g;
tor_inte(3) = 0;

th_inte     = int_e(4)*ctr.gain.ali;

== matlab function controller_v13/Adaptive Controller/observer/External Torque Observer ==
  data: time input; omega input; omega_hat output; torque_x input; torque_y input; ext_torque_hat input; omega_hat input; ext_torque_hat output; ctr parameter; rbt parameter; mdl parameter
function [omega_hat, ext_torque_hat] = fcn(time, omega, torque_x, torque_y, ext_torque_hat, omega_hat, ctr, rbt, mdl)
   
if time > mdl.i_delay
     
    omega_hat = omega_hat(:);
    ext_torque_hat = ext_torque_hat(:);
    ext_torque_hat_xy = ext_torque_hat(1:2);
    J = diag([rbt.ixx, rbt.iyy, rbt.izz]);
    omega_cross_J_omega = cross(omega, J*omega);
    x_hat_curr = diag(ctr.torque_obs.state_scaling)*[omega_hat(:); ext_torque_hat_xy(:)];
    u = diag(ctr.torque_obs.input_scaling)*[torque_x - omega_cross_J_omega(1); torque_y - omega_cross_J_omega(2)];
    y = diag(ctr.torque_obs.meas_scaling)*omega(1:2); 
    x_hat_pred = ctr.torque_obs.A*x_hat_curr + ctr.torque_obs.B(:, 1:2)*u; 
    x_hat_next = diag(ctr.torque_obs.out_scaling)*(x_hat_pred + ctr.torque_obs.L*(y - ctr.torque_obs.C*x_hat_pred));
    omega_hat = x_hat_next(1:2,1);
    ext_torque_hat = [x_hat_next(3:4,1); 0.0];
end

end

== matlab function controller_v13/Measurement manager/safety check system/envelope check ==
  data: x input; en output; y input; z input; ctr parameter
function en  = fcn(x,y,z, ctr)

if abs(x)>ctr.safety.enableZone.xmax || abs(y)>ctr.safety.enableZone.ymax || abs(z)>ctr.safety.enableZone.zmax
    en = 0;
else
    en = 1;
end

end

== matlab function controller_v13/Dynamic Sim/conditioning ==
  data: R_norm_flat output size=9; R input size=9; eu output size=3
function [R_norm_flat, eu]  = fcn(R)
%#codegen
% % this assumes that the matrix is flattened by column
% Rm = [Rin(1:3)./norm(Rin(1:3)),Rin(4:6)./norm(Rin(4:6)),Rin(7:9)./norm(Rin(7:9))];
% % conditioning on orthogonality.
% Rout = [Rm(:,1);Rm(:,2);Rm(:,3)];
R = unflatten_rotm(R);
R_norm = normalize_rotm(R);
R_norm_flat = flatten_rotm(R_norm);

% % euler angles
% euy = asin(min(max(Rm(1,3),-1),1));
% eux = atan2(-Rm(2,3),Rm(3,3));
% euz = atan2(-Rm(1,2),Rm(1,1));
% %euz=acos(min(max(Rm(1,1)/cos(euy),-1),1));
% %eux=acos(min(max(Rm(3,3)/cos(euy),-1),1));

%eu = [eux;euy;euz];
eu = rotm2eul(R_norm, "XYZ")'; % Same format as Vicon
% eu = [ypr(3); ypr(2); ypr(1)];
% not being very careful with singularities.

== matlab function controller_v13/Force//Torque to Trajectory Specs/nominal desired voltage/map_selection ==
  data: hover_map output; time input; mdl parameter; som parameter
function hover_map  = fcn(time, mdl, som)
%#codegen

hover_map = 1;  % during a normal flight
if som.en
    if time > som.t_start + som.t_rise + som.t_acc + som.t_dcc
        hover_map = 1;  % afterwards
    elseif time > som.t_start + som.t_rise
    %elseif time > som.t_start + som.t_rise 
        hover_map = 0;  % 
    end
end

== matlab function controller_v13/Dynamic Sim/rigid body dynamics sim ==
  data: dv output double size=3; mforces input double; dR output double size=9; dw output double size=3; v input; R input; w input; rbt parameter; mdl parameter; disturbance input; rsim parameter
function [dv, dR, dw]  = fcn(mforces,v,R,w,rbt,mdl,disturbance, rsim)
%#codegen

R = unflatten_rotm(R); % R_WB

rbt_A_temp = rbt.A2;
inputs = rbt_A_temp * mforces(:);

thrust = inputs(1);
torque = [inputs(2);inputs(3);inputs(4)];

% Linear acceleration
dv = R*[0; 0; 1]*thrust/rbt.m - [0;0;mdl.g] + disturbance(1:3)/rbt.m - mdl.drag_force.linear*v/rbt.m;

% Angular acceleration
J = diag([rsim.rbt.ixx, rsim.rbt.iyy, rsim.rbt.izz]);
dw = J \ ( (torque) - rsim.rbt.torque_damping*w - cross(w,J*w)+ disturbance(4:6)) ;

% dR1 = R(4:6)*w(3)-R(7:9)*w(2);
% dR2 = R(7:9)*w(1)-R(1:3)*w(3);
% dR3 = R(1:3)*w(2)-R(4:6)*w(1);
% dR = [dR1;dR2;dR3];

% Derivative of a rotation matrix: dot{R_WB} = R_WB * Skew(B_omega)
dR = R*skew(w(:));
dR = flatten_rotm(dR);

end

function ss = skew(vec)
% function ss = skew(vec)
%   The skew function maps a vector in R^3 (or R^1) to its
%   skew symmetric matrix in R^(3x3) (or R^(2x2))

% https://github.com/justinthomas/MATLAB-tools/blob/master/hat.m

switch length(vec)
    
    case 3
        ss = [...
            0, -vec(3), vec(2);...
            vec(3), 0, -vec(1);...
            -vec(2), vec(1), 0];
        
    case 1
        ss = [...
            0, vec; ...
            -vec, 0];
end

end

== matlab function controller_v13/Adaptive Controller/ICRA'23 attitude and thrust MPC controller -> It works/External Torque Observer ==
  data: time input; omega input; omega_hat output; torque_x input; torque_y input; ext_torque_hat input; omega_hat input; ext_torque_hat output; ctr parameter; rbt parameter; mdl parameter
function [omega_hat, ext_torque_hat] = fcn(time, omega, torque_x, torque_y, ext_torque_hat, omega_hat, ctr, rbt, mdl)
   
if time > mdl.i_delay
     
    omega_hat = omega_hat(:);
    ext_torque_hat = ext_torque_hat(:);
    J = diag([rbt.ixx, rbt.iyy, rbt.izz]);
    omega_cross_J_omega = cross(omega, J*omega);
    x_hat_curr = diag(ctr.torque_obs.state_scaling)*[omega_hat(:); ext_torque_hat(:)];
    u = diag(ctr.torque_obs.input_scaling)*[torque_x - omega_cross_J_omega(1); torque_y - omega_cross_J_omega(2)];
    y = diag(ctr.torque_obs.meas_scaling)*omega(1:2); 
    x_hat_pred = ctr.torque_obs.A*x_hat_curr + ctr.torque_obs.B(:, 1:2)*u; 
    x_hat_next = diag(ctr.torque_obs.out_scaling)*(x_hat_pred + ctr.torque_obs.L*(y - ctr.torque_obs.C*x_hat_pred));
    omega_hat = x_hat_next(1:2,1);
    ext_torque_hat = x_hat_next(3:4,1);
end

end

== matlab function controller_v13/Measurement manager/safety check system/voltage check ==
  data: voltage input; en output; ctr parameter
function en  = fcn(voltage, ctr)

if sum(voltage>ctr.safety.volt) > 0
    en = 0;
else
    en = 1;
end

end

== matlab function controller_v13/Measurement manager/envelope//voltage check ==
  data: x input; keep_flying output size=1; y input; z input; ctr parameter
function keep_flying  = fcn(x,y,z,ctr)

if abs(x)>ctr.safety.land.xmax || abs(y)>ctr.safety.land.ymax || abs(z)>ctr.safety.land.zmax
    keep_flying = 0;
% elseif voltage(1) > ctr.safety.land.volt
%     keep_flying = 0;    
else
    keep_flying = 1;
end

end

== matlab function controller_v13/Measurement manager/MATLAB Function ==
  data: keep_flying input; landing_in input; landing_out output size=1; cum_in input; cum_out output size=1; ctr parameter; mdl parameter
function [landing_out, cum_out] = fcn(keep_flying, landing_in, cum_in, ctr, mdl)

if keep_flying == 0
    cum_out = cum_in + mdl.T;
else
    cum_out = 0;
end

if cum_out > ctr.safety.land.T || landing_in == 1
    landing_out = 1;
else 
    landing_out = 0;
end

end

== matlab function controller_v13/Measurement manager/voltage check ==
  data: voltage input; keep_flying output size=1; ctr parameter
function keep_flying  = fcn(voltage, ctr)

% if voltage(1)>ctr.safety.land.volt || voltage(2)>ctr.safety.land.volt || voltage(3)>ctr.safety.land.volt || voltage(4)>ctr.safety.land.volt

if sum(voltage>ctr.safety.land.volt)>0
    keep_flying = 0;
else
    keep_flying = 1;
end

end

== matlab function controller_v13/Measurement manager/safety check system/MATLAB Function ==
  data: keep_flying input; en_in input; en_out output size=1; cum_in input; cum_out output size=1; ctr parameter; mdl parameter
function [en_out, cum_out] = fcn(keep_flying, en_in, cum_in, ctr, mdl)

if keep_flying == 0
    cum_out = cum_in + mdl.T;
else
    cum_out = 0;
end

if cum_out > ctr.safety.T || en_in == 0
    en_out = 0;
else 
    en_out = 1;
end

end

== matlab function controller_v13/MATLAB Function ==
  data: u input; y output
function y = fcn(u)

y = u;

== matlab function controller_v13/Adaptive Controller/ICRA'23 attitude and thrust MPC controller -> It works/PD Atttiude Controller ==
  data: time input; cmd_B_torque output; R input; Omega input; Rd input; Omegad input; tau_ext input; ctr parameter; rbt parameter; mdl parameter; att_e output
function [cmd_B_torque, att_e]   = fcn(time, R, Omega, Rd, Omegad, tau_ext, ctr, rbt, mdl)
%#codegen
% r: curr pos
% r_dot: curr vel
% R: current attitude
% Omega: current body rates
% rd : des pos
% rd_d: des vel
% Rd: desired attitude (rotation matrix)
% Omegad: desired angular velocity


% current attitude
R = get_rotation_matrix(R);     % transform vector in rotation matrix
Omega = Omega(:);
Omegad = Omegad(:);

% desired attitude & angvel
Rd = get_rotation_matrix(Rd);

B_ypr_curr = rotm2eul(R);
B_ypr_des = rotm2eul(Rd);

B_ypr_dot_des = get_euler_derivatives(B_ypr_des, Omegad);
B_ypr_dot_curr = get_euler_derivatives(B_ypr_curr, Omega);
B_ypr_e_dot = (B_ypr_dot_curr - B_ypr_dot_des);
B_rpy_e_dot = [B_ypr_e_dot(3); B_ypr_e_dot(2); B_ypr_e_dot(1)];
disp(B_rpy_e_dot)
disp(Omega - Omegad)

B_ypr_e = B_ypr_curr - B_ypr_des;
B_rpy_e = [B_ypr_e(3); B_ypr_e(2); B_ypr_e(1)];
M = diag(ctr.att_pid_e)*B_rpy_e + diag(ctr.att_pid_e_dot)*B_rpy_e_dot + [tau_ext(1); tau_ext(2); 0.0];

%att_e = eR'*eR; % squared norm of the error
att_e = B_rpy_e(:);
cmd_B_torque = M(:);
end

function R = get_rotation_matrix(R)
    R11 = R(1);
    R12 = R(2);
    R13 = R(3);
    R21 = R(4);
    R22 = R(5);
    R23 = R(6);
    R31 = R(7);
    R32 = R(8);
    R33 = R(9);
    R1 = [R11; R21; R31];     % unit (column) vector
    R2 = [R12; R22; R32];
    R3 = [R13; R23; R33];
    R = [R1, R2, R3];
end

function [B_ypr_dot] = get_euler_derivatives(B_ypr, B_omega)
% https://www.astro.rug.nl/software/kapteyn-beta/_downloads/attitude.pdf
sy = sin(B_ypr(1));
cy = cos(B_ypr(1));
sp = sin(B_ypr(2));
cp = cos(B_ypr(2));
E_zyx = [[0; 0; 1], [-sy; cy; 0.0], [cy*cp; sy*cp; -sp]];
B_ypr_dot = E_zyx\B_omega;

end

== matlab function controller_v13/Adaptive Controller/ICRA'23 attitude and thrust MPC controller -> It works/Pakpong;s atttiude ==
  data: time input; R input; Omega input; Rd input; Omegad input; cmd_B_acc_z input; cmd_B_torque output; ctr parameter; rbt parameter; mdl parameter; att_e output
function [cmd_B_torque, att_e]   = fcn(time, R, Omega, Rd, Omegad, cmd_B_acc_z, ctr, rbt, mdl)
%#codegen

%% init
R11 = R(1);
R12 = R(2);
R13 = R(3);
R21 = R(4);
R22 = R(5);
R23 = R(6);
R31 = R(7);
R32 = R(8);
R33 = R(9);
R1 = [R11; R21; R31];     % unit (column) vector
R2 = [R12; R22; R32];
R3 = [R13; R23; R33];
R = [R1, R2, R3];
wx = Omega(1);
wy = Omega(2);
wz = Omega(3);

e3 = [0; 0; 1];
rd_dd = get_rotation_matrix(Rd)*e3*cmd_B_acc_z;

torque_x = ...
- ctr.gain.at3*( mdl.g*wx) - ...
ctr.gain.at2*( dot(R2,rd_dd) );
torque_x = torque_x*rbt.ixx/mdl.g;

torque_y = ...
- ctr.gain.at3*( mdl.g*wy) - ...
ctr.gain.at2*( dot(R1,-rd_dd) );
torque_y = torque_y*rbt.iyy/mdl.g;

torque_z = 0;           % no yaw control

att_e = -[-dot(R2,rd_dd);dot(R1,rd_dd);0];

cmd_B_torque = [torque_x; torque_y; torque_z];

end

function R = get_rotation_matrix(R)
    R11 = R(1);
    R12 = R(2);
    R13 = R(3);
    R21 = R(4);
    R22 = R(5);
    R23 = R(6);
    R31 = R(7);
    R32 = R(8);
    R33 = R(9);
    R1 = [R11; R21; R31];     % unit (column) vector
    R2 = [R12; R22; R32];
    R3 = [R13; R23; R33];
    R = [R1, R2, R3];

end

== matlab function controller_v13/Adaptive Controller/attitude and thrust MPC controller2/Geometric Attitude Controller ==
  data: time input; torque_x output; R input; Omega input; Rd input; Omegad input; ctr parameter; rbt parameter; torque_y output; torque_z output; mdl parameter; att_e output
function [torque_x, torque_y, torque_z, att_e]   = fcn(time, R, Omega, Rd, Omegad, ctr, rbt, mdl)
%#codegen
% r: curr pos
% r_dot: curr vel
% R: current attitude
% Omega: current body rates
% rd : des pos
% rd_d: des vel
% Rd: desired attitude (rotation matrix)
% Omegad: desired angular velocity


% current attitude
R = get_rotation_matrix(R);     % transform vector in rotation matrix
Omega = Omega(:);

% desired attitude & angvel
Rd = get_rotation_matrix(Rd);
Omegad = Omegad(:);
% Omegad      = [0; 0; 0]; % vee(Rd.'*Rd_1dot);
Omegad_1dot = [0; 0; 0]; % vee(Rd.'*Rd_2dot - hat(Omegad)*hat(Omegad));

% inertia matrix
J = diag([ctr.lee.ixx, ctr.lee.iyy, ctr.lee.izz]);

% attitude and angular velocity errors
eR     = (1/2)*vee(Rd.'*R - R.'*Rd);
eOmega = Omega - R.'*Rd*Omegad;

% desired torque
M = -ctr.lee.kR*eR - ctr.lee.kOmega*eOmega + cross(Omega, J*Omega) ...
  - J*(hat(Omega)*R.'*Rd*Omegad - R.'*Rd*Omegad_1dot);

%att_e = eR'*eR; % squared norm of the error
att_e = eR;

torque_x = M(1);
torque_y = M(2);
torque_z = M(3);

end

function vec = vee(ss)
% function vec = vee(skewsymmetric)
%   The vee function maps a skew-symmetric 
%   matrix to a vector

% https://github.com/justinthomas/MATLAB-tools/blob/master/vee.m

if isa(ss,'sym')
    ss = expand(simplify(ss));
end

switch numel(ss)
    
    case 4
        
        if ~isequal(ss(1,2), -ss(2,1))
            %warning('The provided matrix is not skew symmetric')
        end
        
        vec = ss(1,2);

    case 9

        if ~isequal(ss(3,2),-ss(2,3)) || ~isequal(ss(1,3),-ss(3,1)) || ~isequal(ss(2,1),-ss(1,2))
            %warning('The provided matrix is not skew symmetric.')
            %print(ss)
        end

        vec = [ss(3,2); ss(1,3); ss(2,1)];
end

if isa(ss,'sym')
    vec = simplify(vec);
end

end

function ss = hat(vec)
% function ss = hat(vec)
%   The hat function maps a vector in R^3 (or R^1) to its
%   skew symmetric matrix in R^(3x3) (or R^(2x2))

% https://github.com/justinthomas/MATLAB-tools/blob/master/hat.m

switch length(vec)
    
    case 3
        ss = [...
            0, -vec(3), vec(2);...
            vec(3), 0, -vec(1);...
            -vec(2), vec(1), 0];
        
    case 1
        ss = [...
            0, vec; ...
            -vec, 0];
end

end

function R = get_rotation_matrix(R)
    R11 = R(1);
    R12 = R(2);
    R13 = R(3);
    R21 = R(4);
    R22 = R(5);
    R23 = R(6);
    R31 = R(7);
    R32 = R(8);
    R33 = R(9);
    R1 = [R11; R21; R31];     % unit (column) vector
    R2 = [R12; R22; R32];
    R3 = [R13; R23; R33];
    R = [R1, R2, R3];

end

== matlab function controller_v13/Adaptive Controller/attitude and thrust MPC controller2/MATLAB Function ==
  data: u input; y output
function y = fcn(u)

y = u;
